simulink model "MotorCtrl_FOC_Math"  (R2023b)
settings: Solver=FixedStepDiscrete  StartTime=0.0  StopTime=5  FixedStep=MC_Sim_BaseStep  RelTol=1e-3  EnableMultiTasking=on
values from neighbouring files (symbols this model uses):
  MC_ADC_BitNum = 0.0    [MotorControlDataDictionary_Math.sldd]    (also in MotorControlDataDictionary_Physic.sldd)
  MC_ADC_Offset = 0.0    [MotorControlDataDictionary_Math.sldd]    (also in MotorControlDataDictionary_Physic.sldd)
  MC_ADC_VRef = 1.0    [MotorControlDataDictionary_Math.sldd]    (also in MotorControlDataDictionary_Physic.sldd)
  MC_CSA_Gain = 1.0    [MotorControlDataDictionary_Math.sldd]    (also in MotorControlDataDictionary_Physic.sldd)
  MC_Input_Vdc = 13.5    [MotorControlDataDictionary_Math.sldd]    (also in MotorControlDataDictionary_Physic.sldd)
  MC_MOS_DeadTime = 1.0E-6    [MotorControlDataDictionary_Math.sldd]    (also in MotorControlDataDictionary_Physic.sldd)
  MC_Motor_Mechinal_Damp = 1.0E-5    [MotorControlDataDictionary_Math.sldd]    (also in MotorControlDataDictionary_Physic.sldd)
  MC_Motor_Mechinal_Fric = 0.0    [MotorControlDataDictionary_Math.sldd]    (also in MotorControlDataDictionary_Physic.sldd)
  MC_Motor_Mechinal_Inertia = 0.0103    [MotorControlDataDictionary_Math.sldd]    (also in MotorControlDataDictionary_Physic.sldd)
  MC_Motor_Phi = 0.0059190254913385806    [MotorControlDataDictionary_Math.sldd]    (also in MotorControlDataDictionary_Physic.sldd)
  MC_Motor_Rotor_Pn = 4.0    [MotorControlDataDictionary_Math.sldd]    (also in MotorControlDataDictionary_Physic.sldd)
  MC_Motor_Stator_Ld = 5.6345E-5    [MotorControlDataDictionary_Math.sldd]    (also in MotorControlDataDictionary_Physic.sldd)
  MC_Motor_Stator_Lq = 5.6345E-5    [MotorControlDataDictionary_Math.sldd]    (also in MotorControlDataDictionary_Physic.sldd)
  MC_Motor_Stator_Rs = 0.0286    [MotorControlDataDictionary_Math.sldd]    (also in MotorControlDataDictionary_Physic.sldd)
  MC_Param_CurrentPI_Ki = 0.0071879639914134473    [MotorControlDataDictionary_Math.sldd]    (also in MotorControlDataDictionary_Physic.sldd)
  MC_Param_CurrentPI_Kp = 0.283220860906427    [MotorControlDataDictionary_Math.sldd]    (also in MotorControlDataDictionary_Physic.sldd)
  MC_Param_CurrentPI_UdInteMax = 7.794228634059948    [MotorControlDataDictionary_Math.sldd]    (also in MotorControlDataDictionary_Physic.sldd)
  MC_Param_CurrentPI_UdInteMin = -7.794228634059948    [MotorControlDataDictionary_Math.sldd]    (also in MotorControlDataDictionary_Physic.sldd)
  MC_Param_CurrentPI_UdMax = 7.794228634059948    [MotorControlDataDictionary_Math.sldd]    (also in MotorControlDataDictionary_Physic.sldd)
  MC_Param_CurrentPI_UdMin = -7.794228634059948    [MotorControlDataDictionary_Math.sldd]    (also in MotorControlDataDictionary_Physic.sldd)
  MC_Param_CurrentPI_UqInteMax = 7.794228634059948    [MotorControlDataDictionary_Math.sldd]    (also in MotorControlDataDictionary_Physic.sldd)
  MC_Param_CurrentPI_UqInteMin = -7.794228634059948    [MotorControlDataDictionary_Math.sldd]    (also in MotorControlDataDictionary_Physic.sldd)
  MC_Param_CurrentPI_UqMax = 7.794228634059948    [MotorControlDataDictionary_Math.sldd]    (also in MotorControlDataDictionary_Physic.sldd)
  MC_Param_CurrentPI_UqMin = -7.794228634059948    [MotorControlDataDictionary_Math.sldd]    (also in MotorControlDataDictionary_Physic.sldd)
  MC_Param_Flux_Gamma = 750000.0    [MotorControlDataDictionary_Math.sldd]    (also in MotorControlDataDictionary_Physic.sldd)
  MC_Param_Flux_Lalpha = 5.6345E-5    [MotorControlDataDictionary_Math.sldd]    (also in MotorControlDataDictionary_Physic.sldd)
  MC_Param_Flux_Lbeta = 5.6345E-5    [MotorControlDataDictionary_Math.sldd]    (also in MotorControlDataDictionary_Physic.sldd)
  MC_Param_Flux_Ralpha = 0.0286    [MotorControlDataDictionary_Math.sldd]    (also in MotorControlDataDictionary_Physic.sldd)
  MC_Param_Flux_Rbeta = 0.0286    [MotorControlDataDictionary_Math.sldd]    (also in MotorControlDataDictionary_Physic.sldd)
  MC_Param_Luen_BEMFalpha = -17747.803709290976    [MotorControlDataDictionary_Math.sldd]    (also in MotorControlDataDictionary_Physic.sldd)
  MC_Param_Luen_BEMFbeta = -17747.803709290976    [MotorControlDataDictionary_Math.sldd]    (also in MotorControlDataDictionary_Physic.sldd)
  MC_Param_Luen_BEMFErr = -8.0    [MotorControlDataDictionary_Math.sldd]    (also in MotorControlDataDictionary_Physic.sldd)
  MC_Param_Luen_Currentalpha = -507.58718608572195    [MotorControlDataDictionary_Math.sldd]    (also in MotorControlDataDictionary_Physic.sldd)
  MC_Param_Luen_Currentbeta = -507.58718608572195    [MotorControlDataDictionary_Math.sldd]    (also in MotorControlDataDictionary_Physic.sldd)
  MC_Param_Luen_CurrentErr = -8.0    [MotorControlDataDictionary_Math.sldd]    (also in MotorControlDataDictionary_Physic.sldd)
  MC_Param_Luen_PLL_Ki = 2.3480975196640594    [MotorControlDataDictionary_Math.sldd]    (also in MotorControlDataDictionary_Physic.sldd)
  MC_Param_Luen_PLL_Kp = 153.24842212633141    [MotorControlDataDictionary_Math.sldd]    (also in MotorControlDataDictionary_Physic.sldd)
  MC_Param_Luen_Voltagealpha = 17747.803709290976    [MotorControlDataDictionary_Math.sldd]    (also in MotorControlDataDictionary_Physic.sldd)
  MC_Param_Luen_Voltagebeta = 17747.803709290976    [MotorControlDataDictionary_Math.sldd]    (also in MotorControlDataDictionary_Physic.sldd)
  MC_Param_PhasetoReal = 500.0    [MotorControlDataDictionary_Math.sldd]    (also in MotorControlDataDictionary_Physic.sldd)
  MC_Param_SMO_CoffA = 0.97462064069571386    [MotorControlDataDictionary_Math.sldd]    (also in MotorControlDataDictionary_Physic.sldd)
  MC_Param_SMO_CoffB = 0.88739018546454884    [MotorControlDataDictionary_Math.sldd]    (also in MotorControlDataDictionary_Physic.sldd)
  MC_Param_SpeedCtrl_IdMax = 60.0    [MotorControlDataDictionary_Math.sldd]    (also in MotorControlDataDictionary_Physic.sldd)
  MC_Param_SpeedCtrl_IdMin = -60.0    [MotorControlDataDictionary_Math.sldd]    (also in MotorControlDataDictionary_Physic.sldd)
  MC_Param_SpeedCtrl_IqMax = 60.0    [MotorControlDataDictionary_Math.sldd]    (also in MotorControlDataDictionary_Physic.sldd)
  MC_Param_SpeedCtrl_IqMin = -60.0    [MotorControlDataDictionary_Math.sldd]    (also in MotorControlDataDictionary_Physic.sldd)
  MC_Param_SpeedPI_Ki = 0.57248683633241571    [MotorControlDataDictionary_Math.sldd]    (also in MotorControlDataDictionary_Physic.sldd)
  MC_Param_SpeedPI_Kp = 9.1114109857344836    [MotorControlDataDictionary_Math.sldd]    (also in MotorControlDataDictionary_Physic.sldd)
  MC_Param_SpeedtoTheta = 5.0E-5    [MotorControlDataDictionary_Math.sldd]    (also in MotorControlDataDictionary_Physic.sldd)
  MC_Param_SVPWM_DutyMax = 0.98    [MotorControlDataDictionary_Math.sldd]    (also in MotorControlDataDictionary_Physic.sldd)
  MC_Param_SVPWM_DutyMin = 0.02    [MotorControlDataDictionary_Math.sldd]    (also in MotorControlDataDictionary_Physic.sldd)
  MC_Param_SVPWM_SampleOffset1 = 0.02    [MotorControlDataDictionary_Math.sldd]    (also in MotorControlDataDictionary_Physic.sldd)
  MC_Param_SVPWM_SampleOffset2 = 0.015    [MotorControlDataDictionary_Math.sldd]    (also in MotorControlDataDictionary_Physic.sldd)
  MC_Param_SVPWM_SampleValid = 0.011999999999999999    [MotorControlDataDictionary_Math.sldd]    (also in MotorControlDataDictionary_Physic.sldd)
  MC_Sample_CurrentNoise = 1.0E-15    [MotorControlDataDictionary_Math.sldd]    (also in MotorControlDataDictionary_Physic.sldd)
  MC_Sample_Rs = 0.002    [MotorControlDataDictionary_Math.sldd]    (also in MotorControlDataDictionary_Physic.sldd)
  MC_Sample_VbusNoise = 1.0E-15    [MotorControlDataDictionary_Math.sldd]    (also in MotorControlDataDictionary_Physic.sldd)
  MC_Sim_BaseStep = 5.0E-8    [MotorControlDataDictionary_Math.sldd]    (also in MotorControlDataDictionary_Physic.sldd)
  MC_Sim_HFTStep = 5.0E-5    [MotorControlDataDictionary_Math.sldd]    (also in MotorControlDataDictionary_Physic.sldd)
  MC_Sim_MFTStep = 0.002    [MotorControlDataDictionary_Math.sldd]    (also in MotorControlDataDictionary_Physic.sldd)
libraries: simulink x19, spsVoltageMeasurementLib x2, spsDCVoltageSourceLib x1, spsGroundLib x1, spsPermanentMagnetSynchronousMachineLib x1, spsSeriesRLCBranchLib x1, spsThreePhaseVIMeasurementLib x1, spsUniversalBridgeLib x1, sps_lib x1
(part 1 of 4)
settings Model: DataDictionary=MotorControlDataDictionary_Math.sldd  SimulationMode=accelerator  Creator=YXuan  LastModifiedBy=YXuan
settings SolverCC: AutoInsertRateTranBlk=on
settings OptimizationCC: DefaultParameterBehavior=Inlined  DefaultUnderspecifiedDataType=single  EnhancedBackFolding=on  PassReuseOutputArgsAs=Individual arguments  ZeroExternalMemoryAtStartup=off  ZeroInternalMemoryAtStartup=off  EfficientFloat2IntCast=on  OptimizeBlockOrder=speed  DifferentSizesBufferReuse=on  OptimizationCustomize=off  EfficientTunableParamExpr=on
settings DebuggingCC: ParameterPrecisionLossMsg=none
settings ModelReferenceCC: EnableRefExpFcnMdlSchedulingChecks=on
settings SFSimCC: MATLABDynamicMemAlloc=off
settings RTWCC: Description=Embedded Coder  SystemTargetFile=ert.tlc  GenCodeOnly=on  TemplateMakefile=ert_default_tmf  Toolchain=Microsoft Visual C++ 2022 v17.0 | nmake (64-bit Windows)
settings CodeAppCC: ForceParamTrailComments=on  IgnoreCustomStorageClasses=off  IgnoreTestpoints=on  OperatorAnnotations=on  SimulinkDataObjDesc=on  SFDataObjDesc=on  InsertBlockDesc=on
settings ERTTargetCC: TargetLangStandard=C99 (ISO)  InferredTypesCompatibility=on  GenerateSampleERTMain=on  CombineSignalStateStructs=on  SupportAbsoluteTime=off  SupportNonFinite=off  SupportComplex=off  RemoveDisableFunc=on  InlinedParameterPlacement=NonHierarchical  ERTCustomFileTemplate=example_file_process.tlc

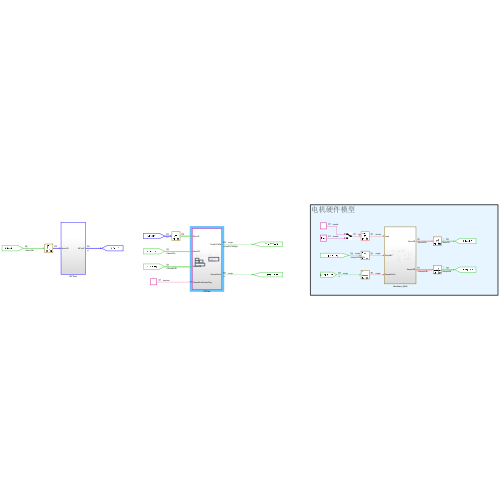
[thumbnail: Simulink's stored preview of the top-level diagram]
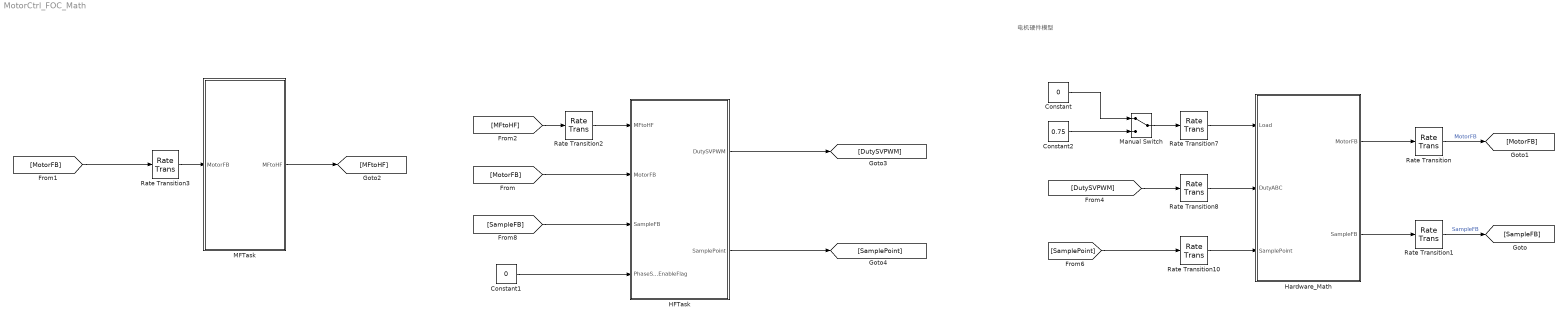
== system MotorCtrl_FOC_Math ==
  note: 电机硬件模型
  Constant : Constant  Value=0
  Constant1 : Constant  Value=0  OutDataTypeStr=boolean
  Constant2 : Constant  Value=0.75
  HFTask : Subsystem  TreatAsAtomicUnit=on  SystemSampleTime=MC_Sim_HFTStep
  Hardware_Math : Subsystem  SystemSampleTime=MC_Sim_BaseStep  VariantControl=MC_Hardware_Motor_Model ==1&MC_Hardware_MotorMOS_Model==1
  MFTask : Subsystem  TreatAsAtomicUnit=on  SystemSampleTime=MC_Sim_MFTStep
  Manual Switch : ManualSwitch
  Rate Transition : RateTransition  OutPortSampleTime=MC_Sim_HFTStep
  Rate Transition1 : RateTransition  OutPortSampleTime=MC_Sim_HFTStep
  Rate Transition10 : RateTransition  OutPortSampleTime=MC_Sim_BaseStep
  Rate Transition2 : RateTransition  OutPortSampleTime=MC_Sim_HFTStep
  Rate Transition3 : RateTransition  OutPortSampleTime=MC_Sim_MFTStep
  Rate Transition7 : RateTransition  OutPortSampleTime=MC_Sim_BaseStep
  Rate Transition8 : RateTransition  OutPortSampleTime=MC_Sim_BaseStep
  wires:
  Hardware_Math/2(SampleFB) -> Rate Transition1/1
  Rate Transition8/1 -> Hardware_Math/2(DutyABC)
  Hardware_Math/1(MotorFB) -> Rate Transition/1
  [SamplePoint] -> Rate Transition10/1
  [DutySVPWM] -> Rate Transition8/1
  Rate Transition1/1 -> [SampleFB]  "SampleFB"
  Rate Transition10/1 -> Hardware_Math/3(SamplePoint)
  Rate Transition7/1 -> Hardware_Math/1(Load)
  Rate Transition/1 -> [MotorFB]  "MotorFB"
  [MotorFB] -> Rate Transition3/1
  MFTask/1(MFtoHF) -> [MFtoHF]
  [MFtoHF] -> Rate Transition2/1
  Constant1/1 -> HFTask/4(PhaseShortEnableFlag)
  [SampleFB] -> HFTask/3(SampleFB)
  [MotorFB] -> HFTask/2(MotorFB)
  HFTask/1(DutySVPWM) -> [DutySVPWM]
  HFTask/2(SamplePoint) -> [SamplePoint]
  Rate Transition2/1 -> HFTask/1(MFtoHF)
  Rate Transition3/1 -> MFTask/1(MotorFB)
  Manual Switch/1 -> Rate Transition7/1
  Constant/1 -> Manual Switch/1
  Constant2/1 -> Manual Switch/2

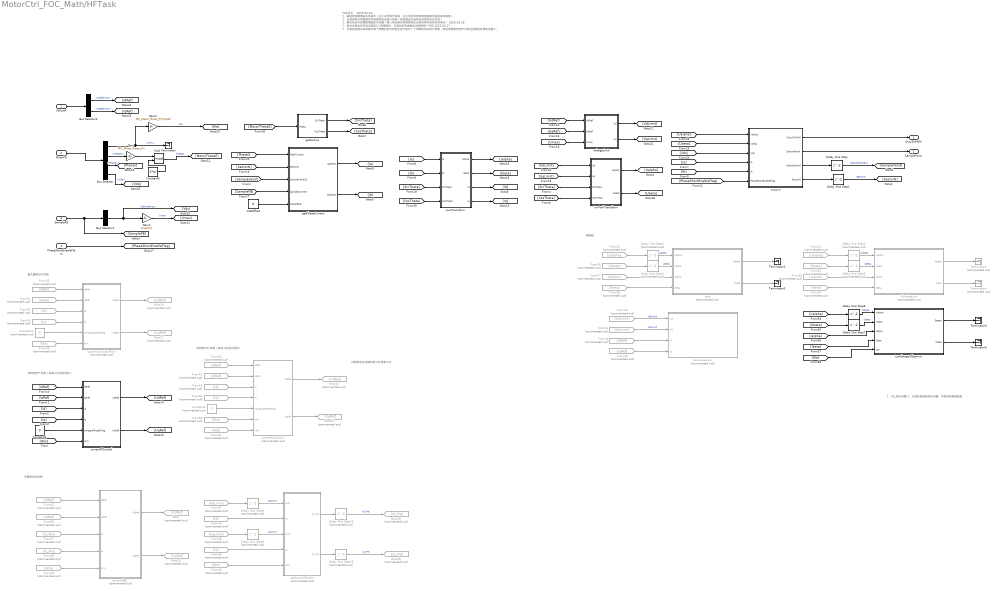
== system MotorCtrl_FOC_Math/HFTask ==
  note: 待更新电压控制的积分抗饱和方式
  note: 传统电流PI控制（前馈+电流抗饱和）
  note: 1、PLL存在问题
      | 2、方程反馈参数存在问题，导致观测角度超前
  note: 观测器
  note: 无差拍电流控制
  note: 开发日志：
      | 2025.03.24:
      | 1、磁链观测器增益应该适中（过小会导致不收敛，过大则会导致观测角度相位超前实际角度）
      | 2、无差拍电流控制是否采用预测电流进行控制？是否要进行旋转反电势的电压补偿？
      | 3、静态电压补偿模型增益如何设置？输入电压是采用理想电压还是采样的电机实际电压？
      | 2025.03.25:
      | 1、测试发现电压和电流呈现2个周期延时，无差拍应考虑做电流预测两个节拍
      | 2025.03.27：
      | 1、无差拍控制应采用延时两个周期的电流和电压进行延时一个周期的电流进行预测，然后用预测电流作为电流控制的反馈电流输入。
  note: 复矢量电流PI控制
  note: 传统电流PI控制（前馈+电压抗饱和）
  MFtoHF : Inport
  MotorFB : Inport  Port=2
  SampleFB : Inport  Port=3
  PhaseShortEnableFlag : Inport  Port=4
  Bus Selector : BusSelector  OutputSignals=Wm,ThetaM,PhaseI,Vdq
  Bus Selector1 : BusSelector  OutputSignals=SampleVus
  Bus Selector3 : BusSelector  OutputSignals=IdRefLimit,IqRefLimit
  CSAOffset : Constant  Value=0  OutDataTypeStr=single
  Constant1 : Constant  Commented=on  Value=0  OutDataTypeStr=boolean
  Constant2 : Constant  Value=0  OutDataTypeStr=boolean
  Constant3 : Constant  Commented=on  Value=0  OutDataTypeStr=boolean
  Constant6 : Constant  Value=2*pi  OutDataTypeStr=single
  Delay One Step{,1,6..7} (4 alike) : Delay
  Delay One Step12 : Delay  Commented=on  DelayLength=0
  Delay One Step13 : Delay  Commented=on  DelayLength=0
  Delay One Step{2..5} (4 alike) : Delay  Commented=on
  Delay One Step8 : Delay  Commented=on  DelayLength=1
  Delay One Step9 : Delay  Commented=on  DelayLength=1
  From25 : From  Commented=on  GotoTag=Ualpha
  From26 : From  Commented=on  GotoTag=Ubeta
  From27 : From  Commented=on  GotoTag=Ialpha
  From28 : From  Commented=on  GotoTag=Ibeta
  From31 : From  Commented=on  GotoTag=Ualpha
  From32 : From  Commented=on  GotoTag=Ubeta
  From33 : From  Commented=on  GotoTag=Ialpha
  From34 : From  Commented=on  GotoTag=Ibeta
  From{35,42,50,60} (4 alike) : From  Commented=on  GotoTag=IdRef
  From{36,43,51,61} (4 alike) : From  Commented=on  GotoTag=IqRef
  From37 : From  Commented=on  GotoTag=Id_Pre
  From38 : From  Commented=on  GotoTag=Iq_Pre
  From39 : From  Commented=on  GotoTag=Wm
  From40 : From  Commented=on  GotoTag=UdLimit
  From41 : From  Commented=on  GotoTag=UqLimit
  From44 : From  Commented=on  GotoTag=Id
  From45 : From  Commented=on  GotoTag=Iq
  From46 : From  Commented=on  GotoTag=Wm
  From47 : From  Commented=on  GotoTag=UdLimit
  From48 : From  Commented=on  GotoTag=UqLimit
  From49 : From  Commented=on  GotoTag=We
  From52 : From  Commented=on  GotoTag=Id
  From53 : From  Commented=on  GotoTag=Iq
  From59 : From  Commented=on  GotoTag=Wm
  From62 : From  Commented=on  GotoTag=Id
  From63 : From  Commented=on  GotoTag=Iq
  From64 : From  Commented=on  GotoTag=Vdq
  Gain : Gain  Gain=MC_Motor_Rotor_Pn  OutDataTypeStr=single
  Gain1 : Gain  Gain=1/sqrt(3)  OutDataTypeStr=single
  Gain2 : Gain  Gain=MC_Motor_Rotor_Pn*pi/30
  Goto : Goto  Commented=on  GotoTag=UdRef
  Goto26 : Goto  Commented=on  GotoTag=UqRef
  Goto27 : Goto  Commented=on  GotoTag=UqRef
  Goto28 : Goto  Commented=on  GotoTag=Id_Pre
  Goto29 : Goto  Commented=on  GotoTag=Iq_Pre
  Goto30 : Goto  Commented=on  GotoTag=UdRef
  Goto31 : Goto  Commented=on  GotoTag=UqRef
  Goto32 : Goto  Commented=on  GotoTag=UdRef
  LuenbergerObservor : Subsystem
  Mod : Math  Operator=mod
  Terminator{,2..3,5..6} (5 alike) : Terminator
  Terminator1 : Terminator  Commented=on
  Terminator4 : Terminator  Commented=on
  axisTransform : Subsystem
  currentComplexPICtrl : Subsystem  Commented=on
  currentDBC : Subsystem  Commented=on
  currentPIControl : Subsystem
  currentPIControl1 : Subsystem  Commented=on
  fluxobservor : Subsystem  Commented=on
  getCurrentPredict : Subsystem  Commented=on
  getPhaseCurrent : Subsystem
  getSinCos : Subsystem
  invParkTransform : Subsystem
  scvmobservor : Subsystem  Commented=on
  smo : Subsystem  Commented=on
  svpwm : Subsystem  TreatAsAtomicUnit=on
  voltageLimit : Subsystem
  DutySVPWM : Outport
  SamplePoint : Outport  Port=2
  wires:
  MFtoHF/1 -> Bus Selector3/1
  Delay One Step2/1 -> smo/1(Valpha)  "Ualpha"
  From25/1 -> Delay One Step2/1
  Delay One Step3/1 -> smo/2(Vbeta)  "Ubeta"
  From26/1 -> Delay One Step3/1
  From27/1 -> smo/3(Ialpha)
  From28/1 -> smo/4(Ibeta)
  smo/1(Speed) -> Terminator2/1
  smo/2(Theta) -> Terminator3/1
  [PhaseShortEnableFlag] -> svpwm/6(PhaseShortEnableFlag)
  [Umax] -> voltageLimit/3(Umax)
  svpwm/4(SectorN) -> Delay One Step1/1
  axisTransform/2(Ibeta) -> [Ibeta]
  svpwm/3(SampleValid) -> Delay One Step/1
  svpwm/1(DutySVPWM) -> DutySVPWM/1
  [SampleFB] -> getPhaseCurrent/4(SampleCurrent)
  [SectorN] -> getPhaseCurrent/2(SectorN)
  [UdRef] -> voltageLimit/1(UdRef)
  [UdLimit] -> invParkTransform/1(Ud)
  currentPIControl/1(UdRef) -> [UdRef]
  [Ubeta] -> svpwm/2(Vbeta)
  axisTransform/1(Ialpha) -> [Ialpha]
  [UqRef] -> voltageLimit/2(UqRef)
  [Ualpha] -> svpwm/1(Valpha)
  [Ia] -> axisTransform/1(Ia)
  svpwm/2(SamplePoint) -> SamplePoint/1
  currentPIControl/2(UqRef) -> [UqRef]
  [Vdc] -> svpwm/3(Vdc)
  voltageLimit/1(Ud) -> [UdLimit]
  [MotorThetaE] -> getSinCos/1(Theta)
  [Id] -> currentPIControl/3(Id)
  getSinCos/1(SinTheta) -> [SinTheta]
  [SampleValid] -> getPhaseCurrent/3(SampleValid[2])
  axisTransform/3(Id) -> [Id]
  getPhaseCurrent/2(Ibselect) -> [Ib]
  [Wm] -> currentPIControl/6(Wm)
  axisTransform/4(Iq) -> [Iq]
  [Iq] -> currentPIControl/4(Iq)
  Constant2/1 -> currentPIControl/5(IntregralResetFlag)
  [Ib] -> axisTransform/2(Ib)
  [UqLimit] -> invParkTransform/2(Uq)
  [SinTheta] -> invParkTransform/3(SinTheta)
  Delay One Step1/1 -> [SectorN]  "SectorN"
  [CosTheta] -> invParkTransform/4(CosTheta)
  [PhaseI] -> getPhaseCurrent/1(RealCurrent)
  invParkTransform/1(Ualpha) -> [Ualpha]
  Delay One Step/1 -> [SampleValid]  "SampleValid[2]"
  getSinCos/2(CosTheta) -> [CosTheta]
  voltageLimit/2(Uq) -> [UqLimit]
  [SinTheta] -> axisTransform/3(SinTheta)
  getPhaseCurrent/1(Iaselect) -> [Ia]
  CSAOffset/1 -> getPhaseCurrent/5(CSAOffset)
  [CosTheta] -> axisTransform/4(CosTheta)
  invParkTransform/2(Ubeta) -> [Ubeta]
  [Ib] -> svpwm/5(Ib)
  [Ia] -> svpwm/4(Ia)
  Bus Selector/2 -> Gain/1  "<ThetaM>"
  PhaseShortEnableFlag/1 -> [PhaseShortEnableFlag]
  Bus Selector/1 -> Terminator/1, Gain2/1  "<Wm>"
  Mod/1 -> [MotorThetaE]  "ThetaE"
  Bus Selector/3 -> [PhaseI]  "<PhaseI>"
  Gain/1 -> Mod/1
  Bus Selector1/1 -> [Vdc], Gain1/1  "<SampleVus>"
  SampleFB/1 -> [SampleFB], Bus Selector1/1
  Gain1/1 -> [Umax]  "Umax"
  Constant6/1 -> Mod/2
  MotorFB/1 -> Bus Selector/1
  Bus Selector3/1 -> [IdRef]  "<IdRefLimit>"
  Bus Selector3/2 -> [IqRef]  "<IqRefLimit>"
  [IdRef] -> currentPIControl/1(IdRef)
  [IqRef] -> currentPIControl/2(IqRef)
  From34/1 -> fluxobservor/4(Ibeta)
  From33/1 -> fluxobservor/3(Ialpha)
  From32/1 -> Delay One Step5/1
  From31/1 -> Delay One Step4/1
  Delay One Step4/1 -> fluxobservor/1(Valpha)  "Ualpha"
  Delay One Step5/1 -> fluxobservor/2(Vbeta)  "Ubeta"
  fluxobservor/1(Speed) -> Terminator1/1
  fluxobservor/2(Theta) -> Terminator4/1
  currentDBC/2(UqRef) -> Goto26/1
  From36/1 -> currentDBC/2(IqRef)
  From35/1 -> currentDBC/1(IdRef)
  From37/1 -> currentDBC/3(Id)
  From38/1 -> currentDBC/4(Iq)
  From39/1 -> currentDBC/5(Wm)
  From41/1 -> scvmobservor/2(Vq)  "UqLimit"
  From40/1 -> scvmobservor/1(Vd)  "UdLimit"
  From42/1 -> scvmobservor/3(Id)
  From43/1 -> scvmobservor/4(Iq)
  Gain2/1 -> [We]  "We"
  From44/1 -> getCurrentPredict/2(Id)
  From45/1 -> getCurrentPredict/4(Iq)
  From46/1 -> getCurrentPredict/5(Wm)
  From47/1 -> Delay One Step8/1
  From48/1 -> Delay One Step9/1
  getCurrentPredict/1(Id_Pre) -> Delay One Step12/1
  getCurrentPredict/2(Iq_Pre) -> Delay One Step13/1
  currentDBC/1(UdRef) -> Goto/1
  Delay One Step8/1 -> getCurrentPredict/1(Ud1)  "UdLimit"
  Delay One Step9/1 -> getCurrentPredict/3(Uq1)  "UqLimit"
  Delay One Step12/1 -> Goto28/1  "Id_Pre"
  Delay One Step13/1 -> Goto29/1  "Iq_Pre"
  From51/1 -> currentComplexPICtrl/2(IqRef)
  From50/1 -> currentComplexPICtrl/1(IdRef)
  Constant1/1 -> currentComplexPICtrl/5(IntregralResetFlag)
  From53/1 -> currentComplexPICtrl/4(Iq)
  From49/1 -> currentComplexPICtrl/6(Wm)
  From52/1 -> currentComplexPICtrl/3(Id)
  currentComplexPICtrl/2(UqRef) -> Goto27/1
  currentComplexPICtrl/1(UdRef) -> Goto30/1
  LuenbergerObservor/1(Speed) -> Terminator5/1
  LuenbergerObservor/2(Theta) -> Terminator6/1
  [Ibeta] -> LuenbergerObservor/4(Ibeta)
  [Ialpha] -> LuenbergerObservor/3(Ialpha)
  [Ubeta] -> Delay One Step7/1
  [Ualpha] -> Delay One Step6/1
  Delay One Step7/1 -> LuenbergerObservor/2(Vbeta)  "Ubeta"
  Delay One Step6/1 -> LuenbergerObservor/1(Valpha)  "Ualpha"
  [We] -> LuenbergerObservor/5(We)
  From61/1 -> currentPIControl1/2(IqRef)
  From60/1 -> currentPIControl1/1(IdRef)
  Constant3/1 -> currentPIControl1/5(IntregralResetFlag)
  From63/1 -> currentPIControl1/4(Iq)
  From59/1 -> currentPIControl1/6(Wm)
  From62/1 -> currentPIControl1/3(Id)
  currentPIControl1/2(UqRef) -> Goto31/1
  currentPIControl1/1(UdRef) -> Goto32/1
  Bus Selector/4 -> [Vdq]  "<Vdq>"
  From64/1 -> currentPIControl1/7(Vdq)

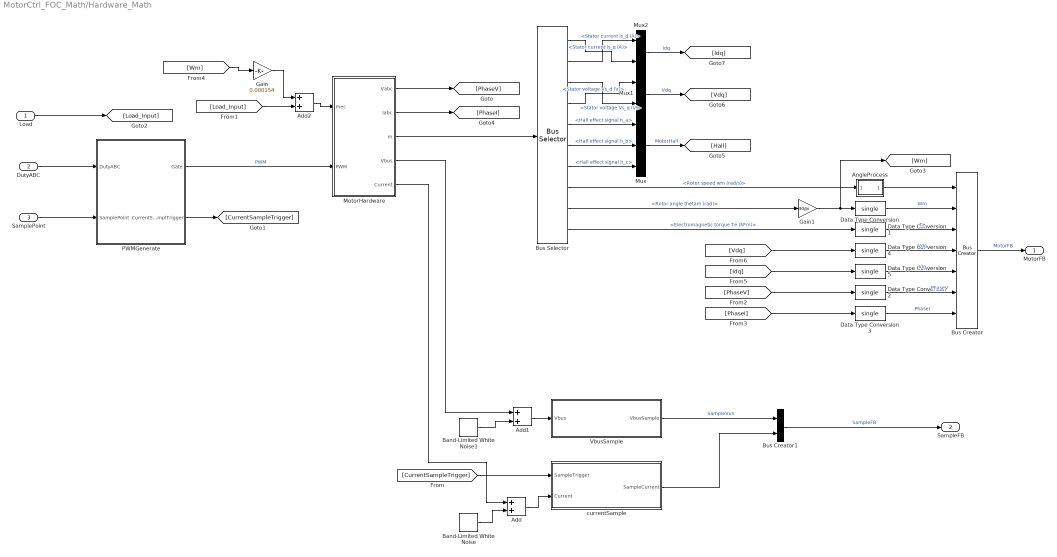
== system MotorCtrl_FOC_Math/Hardware_Math ==
  Load : Inport
  DutyABC : Inport  Port=2
  SamplePoint : Inport  Port=3
  Add : Sum
  Add1 : Sum
  Add2 : Sum
  AngleProcess : Subsystem
  Band-Limited White Noise : simulink/Sources/Band-Limited White Noise  Cov=[MC_Sample_CurrentNoise]  Ts=MC_Sim_BaseStep  seed=[23341]
  Band-Limited White Noise1 : simulink/Sources/Band-Limited White Noise  Cov=[MC_Sample_VbusNoise]  Ts=MC_Sim_BaseStep  seed=[23341]
  Bus Creator : BusCreator  Inputs=7
  Bus Creator1 : BusCreator  Inputs=2
  Bus Selector : BusSelector  OutputSignals=Stator current is_q (A),Stator current is_d (A),Stator voltage Vs_q (V),Stator voltage Vs_d (V),Hall effect signal h_a,Hall effect signal h_b,Hall effect signal h_c,Rotor speed wm (rad/s),Rotor angle thetam (rad),Electromagnetic torque Te (N*m)
  Data Type Conversion{,1..5} (6 alike) : DataTypeConversion  OutDataTypeStr=single  SaturateOnIntegerOverflow=off  RndMeth=Floor
  Gain : Gain  Gain=0.000154
  Gain1 : Gain  Gain=30/pi
  MotorHardware : Subsystem
  Mux : Mux  Inputs=3
  Mux1 : Mux  Inputs=2
  Mux2 : Mux  Inputs=2
  PWMGenerate : Subsystem  SystemSampleTime=MC_Sim_BaseStep
  VbusSample : Subsystem
  currentSample : Subsystem  Variant=on  VariantControl=Subsystem
  MotorFB : Outport
  SampleFB : Outport  Port=2
  wires:
  Band-Limited White Noise/1 -> Add/2
  Add/1 -> currentSample/2(Current)
  Add1/1 -> VbusSample/1(Vbus)
  Band-Limited White Noise1/1 -> Add1/2
  [CurrentSampleTrigger] -> currentSample/1(SampleTrigger)
  PWMGenerate/2(CurrentSamplTrigger) -> [CurrentSampleTrigger]
  DutyABC/1 -> PWMGenerate/1(DutyABC)
  SamplePoint/1 -> PWMGenerate/2(SamplePoint)
  Load/1 -> [Load_Input]
  Gain1/1 -> [Wm], Data Type Conversion/1
  AngleProcess/1(Out1) -> Bus Creator/1
  [PhaseV] -> Data Type Conversion2/1
  [PhaseI] -> Data Type Conversion3/1
  VbusSample/1(VbusSample) -> Bus Creator1/1  "SampleVus"
  currentSample/1(SampleCurrent) -> Bus Creator1/2
  Bus Creator1/1 -> SampleFB/1  "SampleFB"
  PWMGenerate/1(Gate) -> MotorHardware/2(PWM)  "PWM"
  MotorHardware/1(Vabc) -> [PhaseV]
  MotorHardware/2(Iabc) -> [PhaseI]
  MotorHardware/3(m) -> Bus Selector/1
  MotorHardware/5(Current) -> Add/1
  MotorHardware/4(Vbus) -> Add1/1
  Data Type Conversion/1 -> Bus Creator/2  "Wm"
  Data Type Conversion1/1 -> Bus Creator/3  "Te"
  Data Type Conversion2/1 -> Bus Creator/6  "PhaseV"
  Data Type Conversion3/1 -> Bus Creator/7  "PhaseI"
  Bus Creator/1 -> MotorFB/1  "MotorFB"
  Add2/1 -> MotorHardware/1(mec)
  [Load_Input] -> Add2/2
  [Wm] -> Gain/1
  Gain/1 -> Add2/1
  Bus Selector/5 -> Mux/1  "<Hall effect signal h_a>"
  Bus Selector/6 -> Mux/2  "<Hall effect signal h_b>"
  Bus Selector/7 -> Mux/3  "<Hall effect signal h_c>"
  Mux/1 -> [Hall]  "MotorHall"
  Mux1/1 -> [Vdq]  "Vdq"
  Bus Selector/3 -> Mux1/2  "<Stator voltage Vs_q (V)>"
  Bus Selector/4 -> Mux1/1  "<Stator voltage Vs_d (V)>"
  Bus Selector/2 -> Mux2/1  "<Stator current is_d (A)>"
  Bus Selector/1 -> Mux2/2  "<Stator current is_q (A)>"
  Mux2/1 -> [Idq]  "Idq"
  [Vdq] -> Data Type Conversion4/1
  [Idq] -> Data Type Conversion5/1
  Data Type Conversion5/1 -> Bus Creator/5  "Idq"
  Data Type Conversion4/1 -> Bus Creator/4  "Vdq"
  Bus Selector/10 -> Data Type Conversion1/1  "<Electromagnetic torque Te (N*m)>"
  Bus Selector/9 -> Gain1/1  "<Rotor angle thetam (rad)>"
  Bus Selector/8 -> AngleProcess/1(In1)  "<Rotor speed wm (rad/s)>"

== system MotorCtrl_FOC_Math/MFTask ==
  MotorFB : Inport
  Bus Creator : BusCreator  Inputs=2
  Bus Selector : BusSelector  OutputSignals=Wm
  Constant : Constant  Value=1500  OutDataTypeStr=single
  From2 : From  Commented=on  GotoTag=SpeedTarget
  From3 : From  Commented=on  GotoTag=SpeedMotor
  Goto : Goto  Commented=on  GotoTag=IdRef
  Goto1 : Goto  Commented=on  GotoTag=IqRef
  getCurrentLimit : Subsystem
  piofSpeed : Subsystem
  smcofSpeed : Subsystem  Commented=on
  MFtoHF : Outport
  wires:
  MotorFB/1 -> Bus Selector/1
  Bus Selector/1 -> [SpeedMotor]  "<Wm>"
  Bus Creator/1 -> MFtoHF/1
  smcofSpeed/1(IdRef) -> Goto/1
  smcofSpeed/2(IqRef) -> Goto1/1
  piofSpeed/1(IdRef) -> [IdRef]
  piofSpeed/2(IqRef) -> [IqRef]
  getCurrentLimit/2(IqRefLimit) -> [IqRefLimit]
  getCurrentLimit/1(IdRefLimit) -> [IdRefLimit]
  [IdRefLimit] -> Bus Creator/1
  [IqRefLimit] -> Bus Creator/2
  Constant/1 -> [SpeedTarget]  "SpeedTarget"
  From2/1 -> smcofSpeed/1(SpeedTarget)
  From3/1 -> smcofSpeed/2(SpeedReal)
  [IdRef] -> getCurrentLimit/1(IdRef)
  [IqRef] -> getCurrentLimit/2(IqRef)
  [SpeedTarget] -> piofSpeed/1(SpeedTarget)
  [SpeedMotor] -> piofSpeed/2(SpeedReal)

== system MotorCtrl_FOC_Math/HFTask/LuenbergerObservor ==
  Valpha : Inport
  Vbeta : Inport  Port=2
  Ialpha : Inport  Port=3
  Ibeta : Inport  Port=4
  We : Inport  Port=5
  Delay One Step : Delay  DelayLength=1  InitialCondition=single(0)
  Terminator : Terminator
  getE : Subsystem
  getSpeedandTheta : Subsystem
  Speed : Outport
  Theta : Outport  Port=2
  wires:
  getSpeedandTheta/2(Theta) -> Theta/1
  getSpeedandTheta/1(Speed) -> Speed/1
  getE/2(Ebeta) -> getSpeedandTheta/2(Ebeta)
  getE/1(Ealpha) -> getSpeedandTheta/1(Ealpha)
  Ibeta/1 -> getE/4(Ibeta)
  Ialpha/1 -> getE/3(Ialpha)
  Vbeta/1 -> getE/2(Vbeta)
  Valpha/1 -> getE/1(Valpha)
  getSpeedandTheta/3(We) -> Delay One Step/1
  We/1 -> Terminator/1
  Delay One Step/1 -> getE/5(We)

== system MotorCtrl_FOC_Math/HFTask/axisTransform ==
  Ia : Inport
  Ib : Inport  Port=2
  SinTheta : Inport  Port=3
  CosTheta : Inport  Port=4
  Add1 : Sum
  Product{,1..3} (4 alike) : Product
  Signal Copy : SignalConversion  OverrideOpt=off
  Subtract : Sum  Inputs=-+
  a_plus_2b : Sum  Inputs=+++  RndMeth=Simplest  OutDataTypeStr=Inherit: Same as first input
  one_by_sqrt3 : Gain  Gain=1/sqrt(3)  RndMeth=Simplest  OutDataTypeStr=Inherit: Same as input
  Ialpha : Outport
  Ibeta : Outport  Port=2
  Id : Outport  Port=3
  Iq : Outport  Port=4
  wires:
  Product3/1 -> Subtract/2
  Product2/1 -> Subtract/1
  Add1/1 -> Id/1  "Id"
  Subtract/1 -> Iq/1  "Iq"
  Product/1 -> Add1/1
  Product1/1 -> Add1/2
  CosTheta/1 -> Product3/2, Product/2
  SinTheta/1 -> Product2/2, Product1/2
  a_plus_2b/1 -> one_by_sqrt3/1
  one_by_sqrt3/1 -> Ibeta/1, Product3/1, Product1/1  "Ibeta"
  Signal Copy/1 -> Ialpha/1, Product2/1, Product/1  "Ialpha"
  Ia/1 -> a_plus_2b/1, Signal Copy/1
  Ib/1 -> a_plus_2b/3, a_plus_2b/2

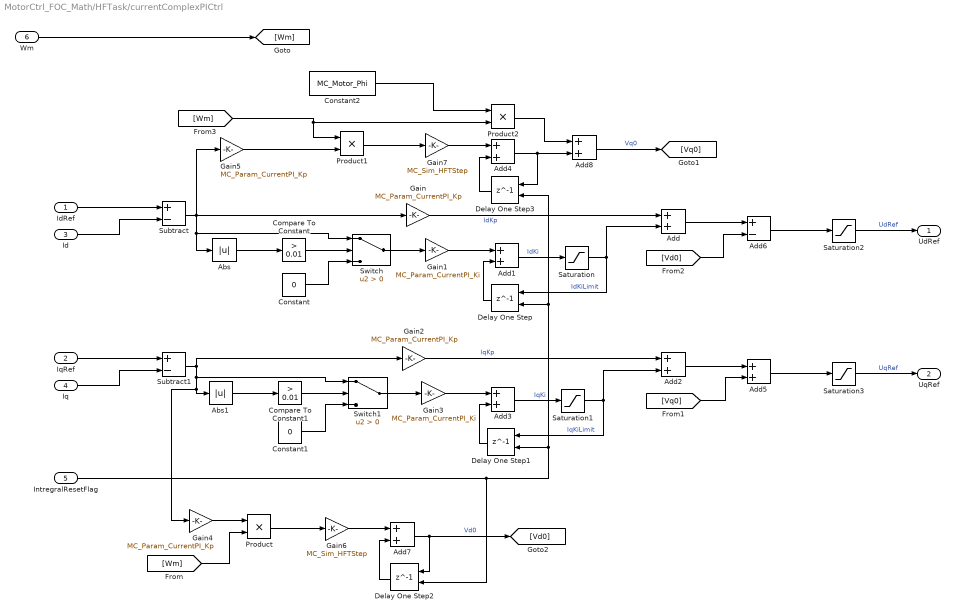
== system MotorCtrl_FOC_Math/HFTask/currentComplexPICtrl ==
  IdRef : Inport
  IqRef : Inport  Port=2
  Id : Inport  Port=3
  Iq : Inport  Port=4
  IntregralResetFlag : Inport  Port=5
  Wm : Inport  Port=6
  Abs : Abs  SaturateOnIntegerOverflow=off
  Abs1 : Abs  SaturateOnIntegerOverflow=off
  Add{,2,5,8} (4 alike) : Sum
  Add{1,3..4,7} (4 alike) : Sum  OutDataTypeStr=single
  Add6 : Sum  Inputs=+-
  Compare To Constant : simulink/Logic and Bit Operations/Compare To Constant  relop=>  const=0.01  OutDataTypeStr=boolean
  Compare To Constant1 : simulink/Logic and Bit Operations/Compare To Constant  relop=>  const=0.01  OutDataTypeStr=boolean
  Constant : Constant  Value=0  OutDataTypeStr=single
  Constant1 : Constant  Value=0  OutDataTypeStr=single
  Constant2 : Constant  Value=MC_Motor_Phi  OutDataTypeStr=single
  Delay One Step{,1..3} (4 alike) : Delay  DelayLength=1  ExternalReset=Level
      settings: InputPortMap=u0,r5
  Gain : Gain  Gain=MC_Param_CurrentPI_Kp  OutDataTypeStr=single
  Gain1 : Gain  Gain=MC_Param_CurrentPI_Ki  OutDataTypeStr=single
  Gain2 : Gain  Gain=MC_Param_CurrentPI_Kp  OutDataTypeStr=single
  Gain3 : Gain  Gain=MC_Param_CurrentPI_Ki  OutDataTypeStr=single
  Gain4 : Gain  Gain=MC_Param_CurrentPI_Kp
  Gain5 : Gain  Gain=MC_Param_CurrentPI_Kp
  Gain6 : Gain  Gain=MC_Sim_HFTStep  OutDataTypeStr=single
  Gain7 : Gain  Gain=MC_Sim_HFTStep  OutDataTypeStr=single
  Product : Product
  Product1 : Product
  Product2 : Product
  Saturation : Saturate  UpperLimit=MC_Param_CurrentPI_UdInteMax  LowerLimit=MC_Param_CurrentPI_UdInteMin
  Saturation1 : Saturate  UpperLimit=MC_Param_CurrentPI_UqInteMax  LowerLimit=MC_Param_CurrentPI_UqInteMin
  Saturation2 : Saturate  UpperLimit=MC_Param_CurrentPI_UdMax  LowerLimit=MC_Param_CurrentPI_UdMin
  Saturation3 : Saturate  UpperLimit=MC_Param_CurrentPI_UqMax  LowerLimit=MC_Param_CurrentPI_UqMin
  Subtract : Sum  Inputs=+-
  Subtract1 : Sum  Inputs=+-
  Switch : Switch  Criteria=u2 > Threshold  SaturateOnIntegerOverflow=off  InputSameDT=off
  Switch1 : Switch  Criteria=u2 > Threshold  SaturateOnIntegerOverflow=off  InputSameDT=off
  UdRef : Outport
  UqRef : Outport  Port=2
  wires:
  Wm/1 -> [Wm]
  Saturation3/1 -> UqRef/1  "UqRef"
  Saturation2/1 -> UdRef/1  "UdRef"
  [Vd0] -> Add6/2
  Add6/1 -> Saturation2/1
  Add/1 -> Add6/1
  [Vq0] -> Add5/2
  Add2/1 -> Add5/1
  [Wm] -> Product/2
  Id/1 -> Subtract/2
  Gain4/1 -> Product/1
  Switch1/1 -> Gain3/1
  Abs1/1 -> Compare To Constant1/1
  Compare To Constant1/1 -> Switch1/2
  Constant1/1 -> Switch1/3
  Constant/1 -> Switch/3
  Compare To Constant/1 -> Switch/2
  Switch/1 -> Gain1/1
  Add5/1 -> Saturation3/1
  IqRef/1 -> Subtract1/1
  Iq/1 -> Subtract1/2
  Subtract1/1 -> Gain2/1, Gain4/1, Abs1/1, Switch1/1
  Gain2/1 -> Add2/1  "IqKp"
  Gain3/1 -> Add3/1
  Delay One Step1/1 -> Add3/2
  Add3/1 -> Saturation1/1  "IqKi"
  Saturation1/1 -> Add2/2, Delay One Step1/1  "IqKiLimit"
  Saturation/1 -> Delay One Step/1, Add/2  "IdKiLimit"
  Add1/1 -> Saturation/1  "IdKi"
  Delay One Step/1 -> Add1/2
  Gain1/1 -> Add1/1
  Abs/1 -> Compare To Constant/1
  Gain/1 -> Add/1  "IdKp"
  Subtract/1 -> Gain5/1, Abs/1, Switch/1, Gain/1
  IdRef/1 -> Subtract/1
  Gain6/1 -> Add7/1
  Product/1 -> Gain6/1
  Delay One Step2/1 -> Add7/2
  Add7/1 -> [Vd0], Delay One Step2/1  "Vd0"
  Add4/1 -> Delay One Step3/1, Add8/2
  Delay One Step3/1 -> Add4/2
  Gain7/1 -> Add4/1
  IntregralResetFlag/1 -> Delay One Step2/2, Delay One Step1/2, Delay One Step3/2, Delay One Step/2
  Product1/1 -> Gain7/1
  Constant2/1 -> Product2/1
  Gain5/1 -> Product1/2
  Add8/1 -> [Vq0]  "Vq0"
  Product2/1 -> Add8/1
  [Wm] -> Product1/1, Product2/2

== system MotorCtrl_FOC_Math/HFTask/currentDBC ==
  note: 无差拍电流控制器（延时1拍）
  IdRef : Inport
  IqRef : Inport  Port=2
  Id : Inport  Port=3
  Iq : Inport  Port=4
  Wm : Inport  Port=5
  Add5 : Sum  Inputs=++-
  Add6 : Sum  Inputs=+++
  Add7 : Sum
  Constant1 : Constant  Value=MC_Motor_Phi  OutDataTypeStr=single
  Gain10 : Gain  Gain=MC_Motor_Stator_Lq
  Gain11 : Gain  Gain=MC_Motor_Stator_Lq/MC_Sim_HFTStep
  Gain12 : Gain  Gain=MC_Motor_Stator_Rs-(MC_Motor_Stator_Lq/MC_Sim_HFTStep)
  Gain13 : Gain  Gain=MC_Motor_Stator_Ld
  Gain8 : Gain  Gain=MC_Motor_Stator_Ld/MC_Sim_HFTStep
  Gain9 : Gain  Gain=MC_Motor_Stator_Rs-(MC_Motor_Stator_Ld/MC_Sim_HFTStep)
  Product2 : Product
  Product3 : Product
  Saturation : Saturate  UpperLimit=MC_Param_CurrentPI_UdMax  LowerLimit=MC_Param_CurrentPI_UdMin
  Saturation1 : Saturate  UpperLimit=MC_Param_CurrentPI_UqMax  LowerLimit=MC_Param_CurrentPI_UqMin
  UdRef : Outport
  UqRef : Outport  Port=2
  wires:
  Wm/1 -> [Wm]
  Iq/1 -> [Iq]
  Id/1 -> [Id]
  IqRef/1 -> [IqRef]
  IdRef/1 -> [IdRef]
  [IdRef] -> Gain8/1
  Gain8/1 -> Add5/1  "IdRef_Vd"
  [Id] -> Gain9/1
  Gain9/1 -> Add5/2  "Id_Vd"
  [Iq] -> Gain10/1
  Gain10/1 -> Product2/2
  [Wm] -> Product2/1
  [IqRef] -> Gain11/1
  Gain11/1 -> Add6/1  "IqRef_Vq"
  Gain12/1 -> Add6/2  "Iq_Vq"
  [Iq] -> Gain12/1
  [Wm] -> Product3/1
  Add7/1 -> Product3/2
  Constant1/1 -> Add7/2
  Gain13/1 -> Add7/1
  [Id] -> Gain13/1
  Saturation/1 -> UdRef/1  "UdRef_DBC"
  Saturation1/1 -> UqRef/1  "UqRef_DBC"
  Add5/1 -> Saturation/1
  Product2/1 -> Add5/3  "Iq_Vd"
  Add6/1 -> Saturation1/1
  Product3/1 -> Add6/3  "Id_Vq"

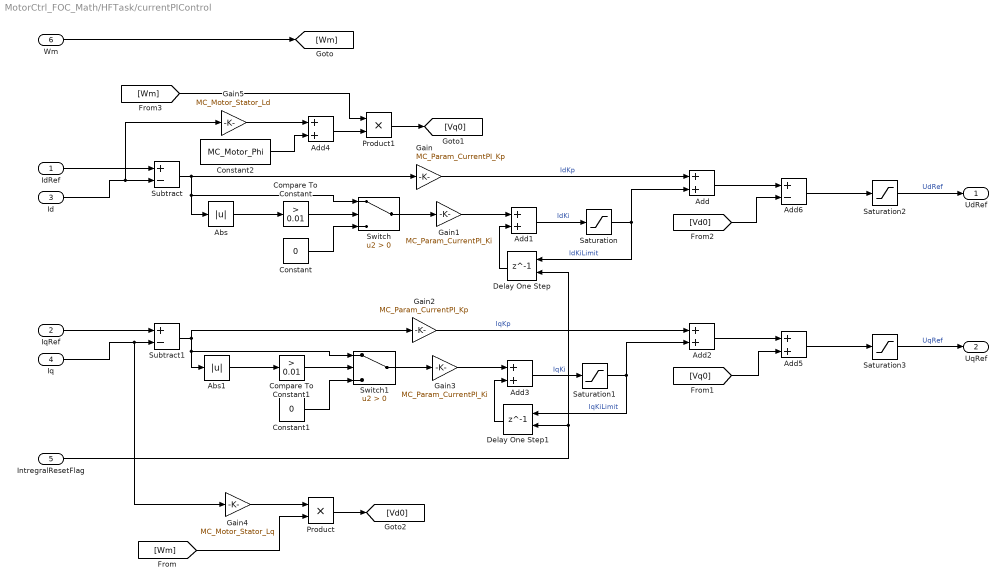
== system MotorCtrl_FOC_Math/HFTask/currentPIControl ==
  IdRef : Inport
  IqRef : Inport  Port=2
  Id : Inport  Port=3
  Iq : Inport  Port=4
  IntregralResetFlag : Inport  Port=5
  Wm : Inport  Port=6
  Abs : Abs  SaturateOnIntegerOverflow=off
  Abs1 : Abs  SaturateOnIntegerOverflow=off
  Add{,2,4..5} (4 alike) : Sum
  Add1 : Sum  OutDataTypeStr=single
  Add3 : Sum  OutDataTypeStr=single
  Add6 : Sum  Inputs=+-
  Compare To Constant : simulink/Logic and Bit Operations/Compare To Constant  relop=>  const=0.01  OutDataTypeStr=boolean
  Compare To Constant1 : simulink/Logic and Bit Operations/Compare To Constant  relop=>  const=0.01  OutDataTypeStr=boolean
  Constant : Constant  Value=0  OutDataTypeStr=single
  Constant1 : Constant  Value=0  OutDataTypeStr=single
  Constant2 : Constant  Value=MC_Motor_Phi  OutDataTypeStr=single
  Delay One Step : Delay  DelayLength=1  ExternalReset=Level
      settings: InputPortMap=u0,r5
  Delay One Step1 : Delay  DelayLength=1  ExternalReset=Level
      settings: InputPortMap=u0,r5
  Gain : Gain  Gain=MC_Param_CurrentPI_Kp  OutDataTypeStr=single
  Gain1 : Gain  Gain=MC_Param_CurrentPI_Ki  OutDataTypeStr=single
  Gain2 : Gain  Gain=MC_Param_CurrentPI_Kp  OutDataTypeStr=single
  Gain3 : Gain  Gain=MC_Param_CurrentPI_Ki  OutDataTypeStr=single
  Gain4 : Gain  Gain=MC_Motor_Stator_Lq
  Gain5 : Gain  Gain=MC_Motor_Stator_Ld
  Product : Product
  Product1 : Product
  Saturation : Saturate  UpperLimit=MC_Param_CurrentPI_UdInteMax  LowerLimit=MC_Param_CurrentPI_UdInteMin
  Saturation1 : Saturate  UpperLimit=MC_Param_CurrentPI_UqInteMax  LowerLimit=MC_Param_CurrentPI_UqInteMin
  Saturation2 : Saturate  UpperLimit=MC_Param_CurrentPI_UdMax  LowerLimit=MC_Param_CurrentPI_UdMin
  Saturation3 : Saturate  UpperLimit=MC_Param_CurrentPI_UqMax  LowerLimit=MC_Param_CurrentPI_UqMin
  Subtract : Sum  Inputs=+-
  Subtract1 : Sum  Inputs=+-
  Switch : Switch  Criteria=u2 > Threshold  SaturateOnIntegerOverflow=off  InputSameDT=off
  Switch1 : Switch  Criteria=u2 > Threshold  SaturateOnIntegerOverflow=off  InputSameDT=off
  UdRef : Outport
  UqRef : Outport  Port=2
  wires:
  IdRef/1 -> Subtract/1
  Subtract/1 -> Gain/1, Switch/1, Abs/1
  Gain/1 -> Add/1  "IdKp"
  Abs/1 -> Compare To Constant/1
  Gain1/1 -> Add1/1
  Delay One Step/1 -> Add1/2
  Add1/1 -> Saturation/1  "IdKi"
  Saturation/1 -> Add/2, Delay One Step/1  "IdKiLimit"
  Saturation1/1 -> Delay One Step1/1, Add2/2  "IqKiLimit"
  Add3/1 -> Saturation1/1  "IqKi"
  Delay One Step1/1 -> Add3/2
  Gain3/1 -> Add3/1
  Gain2/1 -> Add2/1  "IqKp"
  Subtract1/1 -> Switch1/1, Abs1/1, Gain2/1
  Iq/1 -> Gain4/1, Subtract1/2
  IqRef/1 -> Subtract1/1
  IntregralResetFlag/1 -> Delay One Step/2, Delay One Step1/2
  Add5/1 -> Saturation3/1
  Switch/1 -> Gain1/1
  Compare To Constant/1 -> Switch/2
  Constant/1 -> Switch/3
  Constant1/1 -> Switch1/3
  Compare To Constant1/1 -> Switch1/2
  Abs1/1 -> Compare To Constant1/1
  Switch1/1 -> Gain3/1
  Gain4/1 -> Product/1
  Id/1 -> Gain5/1, Subtract/2
  [Wm] -> Product/2
  Gain5/1 -> Add4/1
  Add4/1 -> Product1/2
  Constant2/1 -> Add4/2
  Product1/1 -> [Vq0]
  Product/1 -> [Vd0]
  Add2/1 -> Add5/1
  [Vq0] -> Add5/2
  Add/1 -> Add6/1
  Add6/1 -> Saturation2/1
  [Vd0] -> Add6/2
  Saturation2/1 -> UdRef/1  "UdRef"
  Saturation3/1 -> UqRef/1  "UqRef"
  [Wm] -> Product1/1
  Wm/1 -> [Wm]
